simulink model "twotanks_LQRI"  (R2017b)
settings: Solver=FixedStepAuto  StartTime=0.0  StopTime=150  FixedStep=0.1  RelTol=1e-3
values from neighbouring files (symbols this model uses):
  Ki1 = K1(:,3:4)    [LQRI.m]
  Ki2 = K2(:,3:4)    [LQRI.m]
  Kp1 = K1(:,1:2)    [LQRI.m]
  Kp2 = K2(:,1:2)    [LQRI.m]
libraries: simulink x2
settings Model: Creator=raonymaiafontes  LastModifiedBy=Diogo
settings SolverCC: ZeroCrossAlgorithm=Adaptive
settings DebuggingCC: MaxConsecutiveZCsMsg=none
settings CodeAppCC: StateflowObjectComments=on

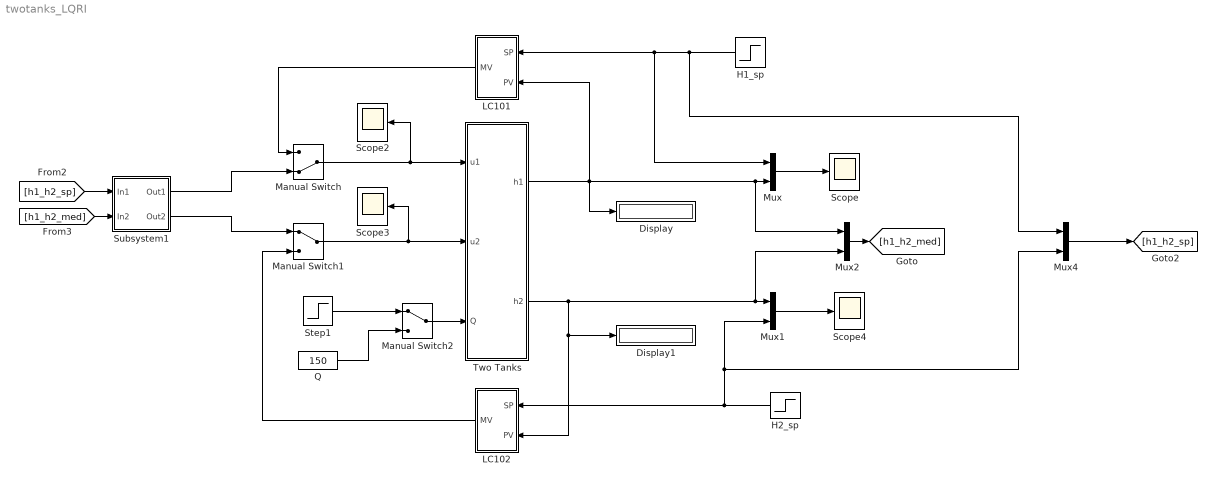
== system twotanks_LQRI ==
  Display : Display
  Display1 : Display
  H1_sp : Step  Time=120  Before=0.65  After=0.35  SampleTime=0
  H2_sp : Step  Time=20  Before=0.28  After=0.678  SampleTime=0
  LC101 : Subsystem
  LC102 : Subsystem
  Manual Switch : ManualSwitch  CurrentSetting=0
  Manual Switch1 : ManualSwitch
  Manual Switch2 : ManualSwitch
  Mux{,1..2,4} (4 alike) : Mux  Inputs=2
  Q : Constant  Value=150
  Scope{,2..4} (4 alike) : Scope
  Step1 : Step  Time=70  Before=150  After=30  SampleTime=0
  Subsystem1 : Subsystem
      mask Display:
      | disp('LQRI')
      | 
      | plot([   -5.0000   -4.9000   -4.8000   -4.7000    -4.6000   -4.5000   -4.4000   -4.3000  -4.2000   -4.1000   -4.0000   -3.9000    -3.8000   -3.7000   -3.6000   -3.5000    -3.4000   -3.3000   -3.2000   -3.1000    -3.0000   -2.9000   -2.8000   -2.7000    -2.6000   -2.5000   -2.4000   -2.3000    -2.2000   -2.1000   -2.0000   -1.9000    -1.8000   -1.7000   -1.6000   -1.5000    -1.4000   -1.3000   -1.2000   -1.1000    -1.0000   -0.9000   -0.8000   -0.7000    -0.6000   -0.5000   -0.4000   -0.3000    -0.2000   -0.1000         0    0.1000     0.2000    0.3000    0.4000    0.5000     0.6000    0.7000    0.8000    0.9000     1.0000    1.1000    1.2000    1.3000     1.4000    1.5000    1.6000    1.7000     1.8000    1.9000    2.0000    2.1000     2.2000    2.3000    2.4000    2.5000     2.6000    2.7000    2.8000    2.9000     3.0000    3.1000    3.2000    3.3000     3.4000    3.5000    3.6000    3.7000     3.8000    3.9000    4.0000    4.1000     4.2000    4.3000    4.4000    4.5000     4.6000    4.7000    4.8000    4.9000     5.0000], [0    0.9950    1.4000    1.7059     1.9596    2.1794    2.3749    2.5515    2.7129    2.8618    3.0000    3.1289    3.2496    3.3630    3.4699    3.5707     3.6661    3.7563    3.8419    3.9230    4.0000    4.0731    4.1425    4.2083    4.2708    4.3301    4.3863    4.4396    4.4900    4.5376    4.5826    4.6249    4.6648    4.7021    4.7371    4.7697    4.8000    4.8280    4.8539    4.8775     4.8990    4.9183    4.9356    4.9508    4.9639    4.9749    4.9840    4.9910    4.9960    4.9990    5.0000    4.9990    4.9960    4.9910    4.9840    4.9749    4.9639    4.9508    4.9356    4.9183    4.8990    4.8775    4.8539    4.8280    4.8000    4.7697    4.7371    4.7021    4.6648    4.6249    4.5826    4.5376    4.4900    4.4396    4.3863    4.3301    4.2708    4.2083    4.1425    4.0731    4.0000    3.9230    3.8419    3.7563    3.6661    3.5707    3.4699    3.3630    3.2496    3.1289    3.0000    2.8618    2.7129    2.5515    2.3749    2.1794     1.9596    1.7059    1.4000    0.9950         0], [   -5.0000   -4.9000   -4.8000   -4.7000    -4.6000   -4.5000   -4.4000   -4.3000  -4.2000   -4.1000   -4.0000   -3.9000    -3.8000   -3.7000   -3.6000   -3.5000    -3.4000   -3.3000   -3.2000   -3.1000    -3.0000   -2.9000   -2.8000   -2.7000    -2.6000   -2.5000   -2.4000   -2.3000    -2.2000   -2.1000   -2.0000   -1.9000    -1.8000   -1.7000   -1.6000   -1.5000    -1.4000   -1.3000   -1.2000   -1.1000    -1.0000   -0.9000   -0.8000   -0.7000    -0.6000   -0.5000   -0.4000   -0.3000    -0.2000   -0.1000         0    0.1000     0.2000    0.3000    0.4000    0.5000     0.6000    0.7000    0.8000    0.9000     1.0000    1.1000    1.2000    1.3000     1.4000    1.5000    1.6000    1.7000     1.8000    1.9000    2.0000    2.1000     2.2000    2.3000    2.4000    2.5000     2.6000    2.7000    2.8000    2.9000     3.0000    3.1000    3.2000    3.3000     3.4000    3.5000    3.6000    3.7000     3.8000    3.9000    4.0000    4.1000     4.2000    4.3000    4.4000    4.5000     4.6000    4.7000    4.8000    4.9000     5.0000], -[0    0.9950    1.4000    1.7059     1.9596    2.1794    2.3749    2.5515    2.7129    2.8618    3.0000    3.1289    3.2496    3.3630    3.4699    3.5707     3.6661    3.7563    3.8419    3.9230    4.0000    4.0731    4.1425    4.2083    4.2708    4.3301    4.3863    4.4396    4.4900    4.5376    4.5826    4.6249    4.6648    4.7021    4.7371    4.7697    4.8000    4.8280    4.8539    4.8775     4.8990    4.9183    4.9356    4.9508    4.9639    4.9749    4.9840    4.9910    4.9960    4.9990    5.0000    4.9990    4.9960    4.9910    4.9840    4.9749    4.9639    4.9508    4.9356    4.9183    4.8990    4.8775    4.8539    4.8280    4.8000    4.7697    4.7371    4.7021    4.6648    4.6249    4.5826    4.5376    4.4900    4.4396    4.3863    4.3301    4.2708    4.2083    4.1425    4.0731    4.0000    3.9230    3.8419    3.7563    3.6661    3.5707    3.4699    3.3630    3.2496    3.1289    3.0000    2.8618    2.7129    2.5515    2.3749    2.1794     1.9596    1.7059    1.4000    0.9950         0])
  Two Tanks : Subsystem
  wires:
  Manual Switch/1 -> Scope2/1, Two Tanks/1(u1)
  LC101/1(MV) -> Manual Switch/1
  Manual Switch1/1 -> Scope3/1, Two Tanks/2(u2)
  LC102/1(MV) -> Manual Switch1/2
  Manual Switch2/1 -> Two Tanks/3(Q)
  Step1/1 -> Manual Switch2/1
  Q/1 -> Manual Switch2/2
  Mux/1 -> Scope/1
  Mux1/1 -> Scope4/1
  Mux2/1 -> [h1_h2_med]
  Mux4/1 -> [h1_h2_sp]
  [h1_h2_sp] -> Subsystem1/1(In1)
  [h1_h2_med] -> Subsystem1/2(In2)
  Two Tanks/1(h1) -> Mux2/1, Mux/2, LC101/2(PV), Display/1
  Two Tanks/2(h2) -> LC102/2(PV), Display1/1, Mux2/2, Mux1/1
  H2_sp/1 -> Mux4/2, Mux1/2, LC102/1(SP)
  H1_sp/1 -> Mux4/1, Mux/1, LC101/1(SP)
  Subsystem1/1(Out1) -> Manual Switch/2
  Subsystem1/2(Out2) -> Manual Switch1/1

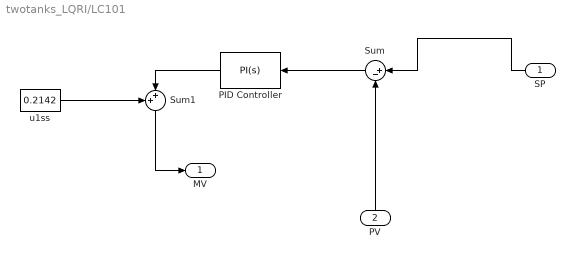
== system twotanks_LQRI/LC101 ==
  SP : Inport
  PV : Inport  Port=2
  PID Controller : simulink/Continuous/PID Controller  Controller=PI  TimeDomain=Continuous-time  SampleTime=-1  IntegratorMethod=Forward Euler  FilterMethod=Forward Euler  Form=Ideal  UseFilter=on  ControllerParametersSource=internal  P=-0.667562978885468  I=0.0981942038508327  D=0  N=100  InitialConditionSource=internal  InitialConditionForIntegrator=0  InitialConditionForFilter=0  ExternalReset=none  LimitOutput=on  UpperSaturationLimit=0.7358  LowerSaturationLimit=-0.2042  LinearizeAsGain=on  AntiWindupMode=back-calculation  Kb=1  TrackingMode=off  Kt=1  PParamMin=[]  PParamMax=[]  IParamMin=[]  IParamMax=[]  DParamMin=[]  DParamMax=[]  NParamMin=[]  NParamMax=[]  KbParamMin=[]  KbParamMax=[]  KtParamMin=[]  KtParamMax=[]  POutMin=[]  POutMax=[]  IOutMin=[]  IOutMax=[]  DOutMin=[]  DOutMax=[]  NOutMin=[]  NOutMax=[]  KbOutMin=[]  KbOutMax=[]  KtOutMin=[]  KtOutMax=[]  IntegratorOutMin=[]  IntegratorOutMax=[]  FilterOutMin=[]  FilterOutMax=[]  SumOutMin=[]  SumOutMax=[]  SumI1OutMin=[]  SumI1OutMax=[]  SumI2OutMin=[]  SumI2OutMax=[]  SumI3OutMin=[]  SumI3OutMax=[]  SumDOutMin=[]  SumDOutMax=[]  SaturationOutMin=[]  SaturationOutMax=[]  IntegratorContinuousStateAttributes=''  IntegratorStateMustResolveToSignalObject=off  IntegratorRTWStateStorageClass=Auto  FilterContinuousStateAttributes=''  FilterStateMustResolveToSignalObject=off  FilterRTWStateStorageClass=Auto  DifferentiatorICPrevScaledInput=0  DifferentiatorOutMin=[]  DifferentiatorOutMax=[]  InitialConditionSetting=State (most efficient)  FilterDiffOutCoefMin=[]  FilterDiffOutCoefMax=[]  SumDenOutMin=[]  SumDenOutMax=[]  SumNumOutMin=[]  SumNumOutMax=[]  ReciprocalOutMin=[]  ReciprocalOutMax=[]  DivideOutMin=[]  DivideOutMax=[]  TunerSelectOption=Transfer Function Based (PID Tuner App)
  Sum : Sum  Inputs=|+-
  Sum1 : Sum  Inputs=++|
  u1ss : Constant  Value=0.2142
  MV : Outport
  wires:
  Sum1/1 -> MV/1
  PV/1 -> Sum/2
  PID Controller/1 -> Sum1/2
  SP/1 -> Sum/1
  u1ss/1 -> Sum1/1
  Sum/1 -> PID Controller/1

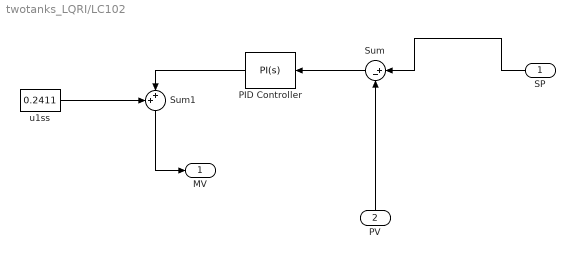
== system twotanks_LQRI/LC102 ==
  SP : Inport
  PV : Inport  Port=2
  PID Controller : simulink/Continuous/PID Controller  Controller=PI  TimeDomain=Continuous-time  SampleTime=-1  IntegratorMethod=Forward Euler  FilterMethod=Forward Euler  Form=Ideal  UseFilter=on  ControllerParametersSource=internal  P=-0.11544378631374  I=6.6123973931149  D=0  N=100  InitialConditionSource=internal  InitialConditionForIntegrator=0  InitialConditionForFilter=0  ExternalReset=none  LimitOutput=on  UpperSaturationLimit=0.95-0.2411  LowerSaturationLimit=0.01-0.2411  LinearizeAsGain=on  AntiWindupMode=back-calculation  Kb=1  TrackingMode=off  Kt=1  PParamMin=[]  PParamMax=[]  IParamMin=[]  IParamMax=[]  DParamMin=[]  DParamMax=[]  NParamMin=[]  NParamMax=[]  KbParamMin=[]  KbParamMax=[]  KtParamMin=[]  KtParamMax=[]  POutMin=[]  POutMax=[]  IOutMin=[]  IOutMax=[]  DOutMin=[]  DOutMax=[]  NOutMin=[]  NOutMax=[]  KbOutMin=[]  KbOutMax=[]  KtOutMin=[]  KtOutMax=[]  IntegratorOutMin=[]  IntegratorOutMax=[]  FilterOutMin=[]  FilterOutMax=[]  SumOutMin=[]  SumOutMax=[]  SumI1OutMin=[]  SumI1OutMax=[]  SumI2OutMin=[]  SumI2OutMax=[]  SumI3OutMin=[]  SumI3OutMax=[]  SumDOutMin=[]  SumDOutMax=[]  SaturationOutMin=[]  SaturationOutMax=[]  IntegratorContinuousStateAttributes=''  IntegratorStateMustResolveToSignalObject=off  IntegratorRTWStateStorageClass=Auto  FilterContinuousStateAttributes=''  FilterStateMustResolveToSignalObject=off  FilterRTWStateStorageClass=Auto  DifferentiatorICPrevScaledInput=0  DifferentiatorOutMin=[]  DifferentiatorOutMax=[]  InitialConditionSetting=State (most efficient)  FilterDiffOutCoefMin=[]  FilterDiffOutCoefMax=[]  SumDenOutMin=[]  SumDenOutMax=[]  SumNumOutMin=[]  SumNumOutMax=[]  ReciprocalOutMin=[]  ReciprocalOutMax=[]  DivideOutMin=[]  DivideOutMax=[]  TunerSelectOption=Transfer Function Based (PID Tuner App)
  Sum : Sum  Inputs=|+-
  Sum1 : Sum  Inputs=++|
  u1ss : Constant  Value=0.2411
  MV : Outport
  wires:
  Sum/1 -> PID Controller/1
  u1ss/1 -> Sum1/1
  SP/1 -> Sum/1
  PID Controller/1 -> Sum1/2
  PV/1 -> Sum/2
  Sum1/1 -> MV/1

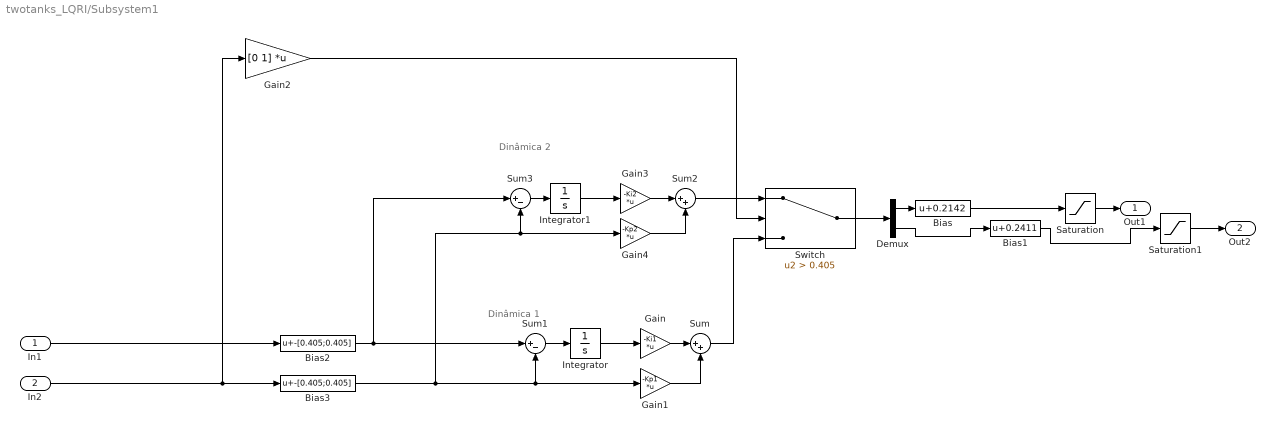
== system twotanks_LQRI/Subsystem1 ==
  note: Dinâmica 1
  note: Dinâmica 2
  In1 : Inport
  In2 : Inport  Port=2
  Bias : Bias  Bias=0.2142
  Bias1 : Bias  Bias=0.2411
  Bias2 : Bias  Bias=-[0.405;0.405]
  Bias3 : Bias  Bias=-[0.405;0.405]
  Demux : Demux  Outputs=2
  Gain : Gain  Gain=-Ki1  Multiplication=Matrix(K*u)
  Gain1 : Gain  Gain=-Kp1  Multiplication=Matrix(K*u)
  Gain2 : Gain  Gain=[0 1]  Multiplication=Matrix(K*u)
  Gain3 : Gain  Gain=-Ki2  Multiplication=Matrix(K*u)
  Gain4 : Gain  Gain=-Kp2  Multiplication=Matrix(K*u)
  Integrator : Integrator
  Integrator1 : Integrator
  Saturation : Saturate  UpperLimit=0.95  LowerLimit=0.01
  Saturation1 : Saturate  UpperLimit=0.95  LowerLimit=0.01
  Sum : Sum  Inputs=|++
  Sum1 : Sum  Inputs=|+-
  Sum2 : Sum  Inputs=|++
  Sum3 : Sum  Inputs=|+-
  Switch : Switch  Criteria=u2 > Threshold  Threshold=0.405
  Out1 : Outport
  Out2 : Outport  Port=2
  wires:
  Bias3/1 -> Gain4/1, Sum3/2, Gain1/1, Sum1/2
  Bias1/1 -> Saturation1/1
  Bias/1 -> Saturation/1
  Demux/1 -> Bias/1
  Saturation1/1 -> Out2/1
  Saturation/1 -> Out1/1
  Demux/2 -> Bias1/1
  Switch/1 -> Demux/1
  Gain3/1 -> Sum2/1
  Integrator1/1 -> Gain3/1
  Gain4/1 -> Sum2/2
  Sum2/1 -> Switch/1
  Sum3/1 -> Integrator1/1
  In1/1 -> Bias2/1
  In2/1 -> Bias3/1, Gain2/1
  Gain2/1 -> Switch/2
  Bias2/1 -> Sum1/1, Sum3/1
  Sum1/1 -> Integrator/1
  Sum/1 -> Switch/3
  Gain1/1 -> Sum/2
  Integrator/1 -> Gain/1
  Gain/1 -> Sum/1

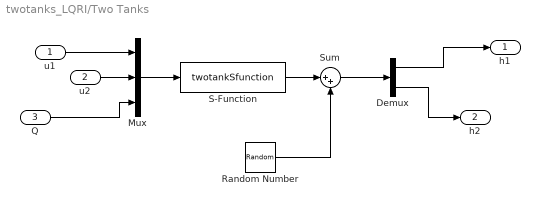
== system twotanks_LQRI/Two Tanks ==
  u1 : Inport
  u2 : Inport  Port=2
  Q : Inport  Port=3
  Demux : Demux  Outputs=2
  Mux : Mux  Inputs=3
  Random Number : RandomNumber  Variance=1e-5  SampleTime=0.1
  S-Function : S-Function  FunctionName=twotankSfunction  SFunctionDeploymentMode=off  EnableBusSupport=off
  Sum : Sum  Inputs=|++
  h1 : Outport
  h2 : Outport  Port=2
  wires:
  u2/1 -> Mux/2
  Q/1 -> Mux/3
  Demux/2 -> h2/1
  u1/1 -> Mux/1
  Demux/1 -> h1/1
  Mux/1 -> S-Function/1
  S-Function/1 -> Sum/1
  Sum/1 -> Demux/1
  Random Number/1 -> Sum/2
